simulink model "Part4_1_Q1sys"  (R2022a)
settings: Solver=VariableStepAuto  StartTime=0.0  StopTime=2000  RelTol=1e-3
settings Model: Creator=theod  LastModifiedBy=theod
settings DebuggingCC: UnconnectedInputMsg=warning  UnconnectedOutputMsg=warning  UnconnectedLineMsg=warning
settings RTWCC: DLArmComputeVersion=19.05

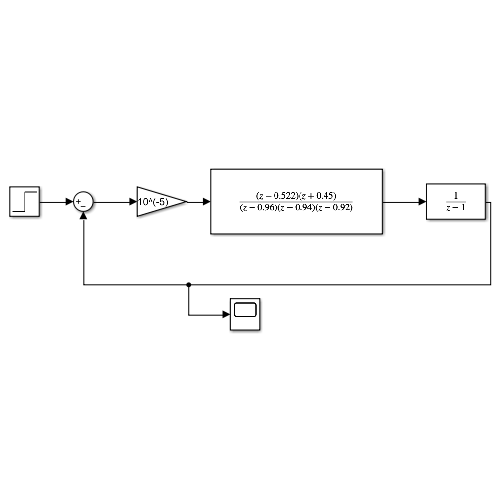
[thumbnail: Simulink's stored preview of the top-level diagram]
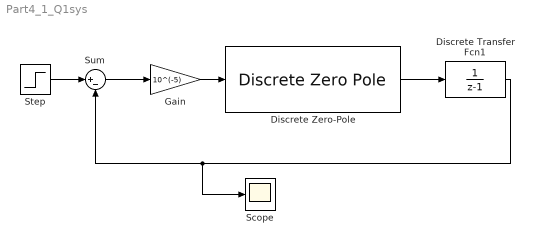
== system Part4_1_Q1sys ==
  Discrete Transfer Fcn1 : DiscreteTransferFcn  Denominator=[1 -1]
  Discrete Zero-Pole : DiscreteZeroPole  Zeros=[0.522 -0.45]  Poles=[0.96 0.94 0.92]  Gain=1  SampleTime=-1
  Gain : Gain  Gain=10^(-5)
  Scope : Scope
  Step : Step  SampleTime=0.1
  Sum : Sum  Inputs=|+-
  wires:
  Discrete Transfer Fcn1/1 -> Scope/1, Sum/2
  Step/1 -> Sum/1
  Sum/1 -> Gain/1
  Gain/1 -> Discrete Zero-Pole/1
  Discrete Zero-Pole/1 -> Discrete Transfer Fcn1/1
